simulink model "Example_Event_Separation_OB_Undirected"  (R2021b)
settings: Solver=FixedStepAuto  StartTime=0.0  StopTime=30  FixedStep=0.0001  RelTol=1e-3  EnableMultiTasking=on
values from neighbouring files (symbols this model uses):
  A = [0  1  0 ... (first row only)    [Event_Separation_OB_Undirected.m]
  ADJ = [0 1 0 0 1 0 ... (first row only)    [Event_Separation_OB_Undirected.m]
  BB = [0  0  1  0  1  0]*0    [Event_Separation_OB_Undirected.m]
  Bu = [0;0;1]    [Event_Separation_OB_Undirected.m]
  c = 1/lambda1    [Event_Separation_OB_Undirected.m]
  Cy = [1 0 0]    [Event_Separation_OB_Undirected.m]
  delta = 0.9*min(min(abs(eig(Q)))/max(abs(eig(P))),min(alpha))    [Event_Separation_OB_Undirected.m]
  F = -P*Cy'    [Event_Separation_OB_Undirected.m]
  K = -Bu'*P    [Event_Separation_OB_Undirected.m]
  LL = diag(sum(ADJ,2))-ADJ    [Event_Separation_OB_Undirected.m]
  nr = nx    [Event_Separation_OB_Undirected.m]
  nx = size(A,1)    [Event_Separation_OB_Undirected.m]
  ny = size(Cy,1)    [Event_Separation_OB_Undirected.m]
  Tc = linspace(0.11,0.16,6)    [Event_Separation_OB_Undirected.m]
  Th = 10    [Event_Separation_OB_Undirected.m]
  theta = 1    [Event_Separation_OB_Undirected.m]
  x0 = x_leader.Data    [Event_Separation_OB_Undirected.m]    (also in x0.mat = [-1.58875392951 1.07389213768 -3.08254744538 2.38426839977 -)
  x0_leader = [1 1 1]    [Event_Separation_OB_Undirected.m]
undefined symbols (not defined in the file or in its folder): Kri_m_Krj_1, Kri_m_Krj_2, Kri_m_Krj_3, Kri_m_Krj_4, Kri_m_Krj_5, Kri_m_Krj_6, ty0_1, ty0_2, ty0_3, ty0_4, ty0_5, ty0_6
settings Model: PauseTimes=0.9999  Creator=Xianwei  LastModifiedBy=kangge648
settings SolverCC: AlgebraicLoopSolver=LineSearch
settings DataIOCC: LimitDataPoints=on  ReturnWorkspaceOutputs=off
settings OptimizationCC: LifeSpan=inf
settings DebuggingCC: AllowSymbolicDim=off  SFUnexpectedBacktrackingDiag=warning  SFNoUnconditionalDefaultTransitionDiag=warning  SFExecutionAtInitializationDiag=none  SFMachineParentedDataDiag=warning  ArithmeticOperatorsInVariantConditions=warning
settings ModelReferenceCC: PropagateSignalLabelsOutOfModel=off
settings SFSimCC: SimUseLocalCustomCode=off  CustomCodeUndefinedFunction=UseInterfaceOnly
settings RTWCC: RTWUseLocalCustomCode=off
settings CodeAppCC: StateflowObjectComments=on
settings GRTTargetCC: TargetLangStandard=C89/C90 (ANSI)
settings ConfigComp: CovMetricSettings=dw  CovSaveCumulativeToWorkspaceVar=on  CovSaveSingleToWorkspaceVar=on  CovExternalEMLEnable=off

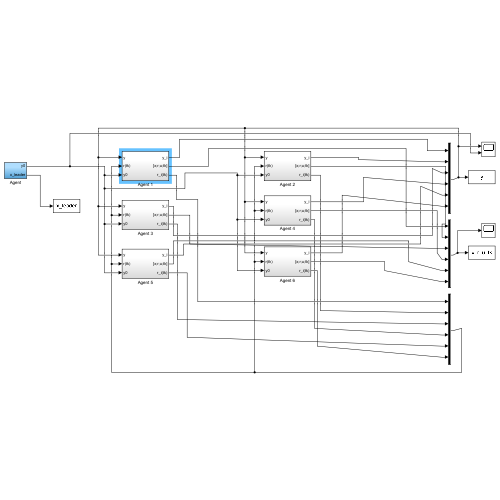
[thumbnail: Simulink's stored preview of the top-level diagram]
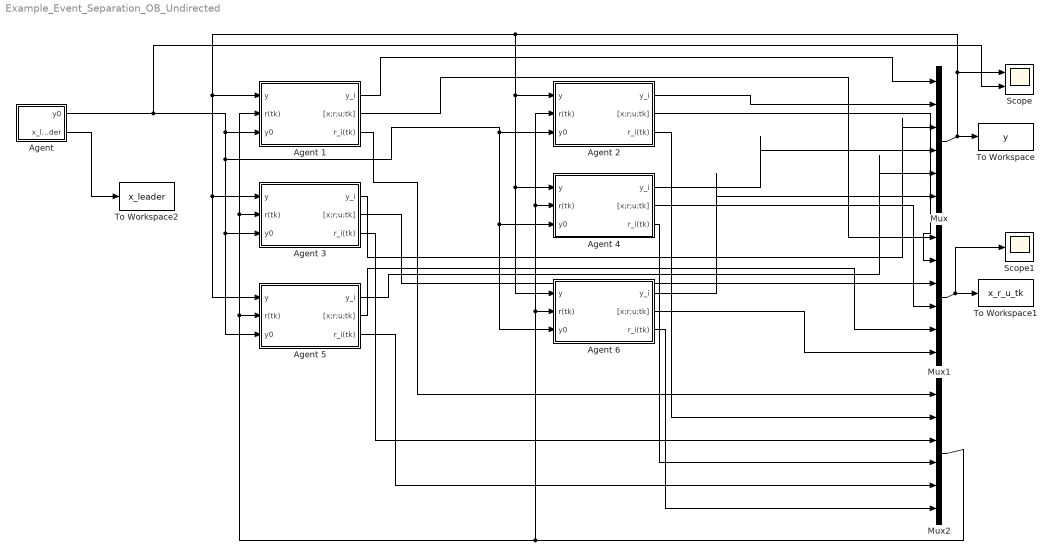
== system Example_Event_Separation_OB_Undirected ==
  Agent : Subsystem
  Agent 1 : Subsystem
  Agent 2 : Subsystem
  Agent 3 : Subsystem
  Agent 4 : Subsystem
  Agent 5 : Subsystem
  Agent 6 : Subsystem
  Mux : Mux  Inputs=6
  Mux1 : Mux  Inputs=6
  Mux2 : Mux  Inputs=6
  Scope : Scope  NumInputPorts=2
  Scope1 : Scope
  To Workspace : ToWorkspace  VariableName=y  SaveFormat=Timeseries  SampleTime=-1
  To Workspace1 : ToWorkspace  VariableName=x_r_u_tk  SaveFormat=Timeseries  SampleTime=-1
  To Workspace2 : ToWorkspace  VariableName=x_leader  SaveFormat=Timeseries  SampleTime=-1
  wires:
  Mux1/1 -> Scope1/1, To Workspace1/1
  Agent 1/1(y_i) -> Mux/1
  Agent 2/1(y_i) -> Mux/2
  Agent 3/1(y_i) -> Mux/3
  Agent 4/1(y_i) -> Mux/4
  Agent 5/1(y_i) -> Mux/5
  Agent 1/2("[x;r;u;tk]") -> Mux1/1
  Agent 2/2("[x;r;u;tk]") -> Mux1/2
  Agent 3/2("[x;r;u;tk]") -> Mux1/3
  Agent 4/2("[x;r;u;tk]") -> Mux1/4
  Agent 5/2("[x;r;u;tk]") -> Mux1/5
  Agent 1/3(r_i(tk)) -> Mux2/1
  Agent 2/3(r_i(tk)) -> Mux2/2
  Agent 3/3(r_i(tk)) -> Mux2/3
  Agent 4/3(r_i(tk)) -> Mux2/4
  Agent 5/3(r_i(tk)) -> Mux2/5
  Agent 6/3(r_i(tk)) -> Mux2/6
  Agent 6/1(y_i) -> Mux/6
  Agent 6/2("[x;r;u;tk]") -> Mux1/6
  Mux/1 -> Agent 5/1(y), Agent 3/1(y), Agent 1/1(y), Agent 6/1(y), Agent 4/1(y), Agent 2/1(y), Scope/1, To Workspace/1
  Mux2/1 -> Agent 5/2(r(tk)), Agent 3/2(r(tk)), Agent 1/2(r(tk)), Agent 6/2(r(tk)), Agent 4/2(r(tk)), Agent 2/2(r(tk))
  Agent/1(y0) -> Scope/2, Agent 6/3(y0), Agent 4/3(y0), Agent 2/3(y0), Agent 5/3(y0), Agent 3/3(y0), Agent 1/3(y0)
  Agent/2(x_leader) -> To Workspace2/1

== system Example_Event_Separation_OB_Undirected/Agent ==
  A : Gain  Gain=A  Multiplication=Matrix(K*u)
  Cy : Gain  Gain=Cy  Multiplication=Matrix(K*u)
  Integrator : Integrator  InitialCondition=x0_leader  ContinuousStateAttributes='x1'
  y0 : Outport
  x_leader : Outport  Port=2
  wires:
  Integrator/1 -> x_leader/1, A/1, Cy/1
  A/1 -> Integrator/1
  Cy/1 -> y0/1

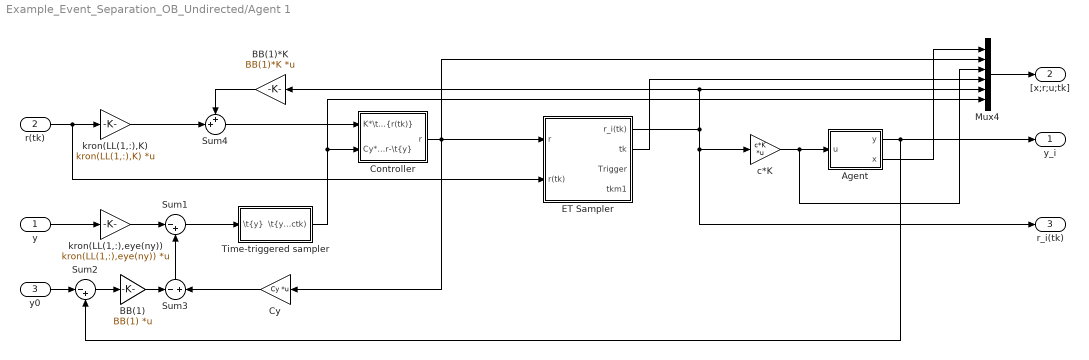
== system Example_Event_Separation_OB_Undirected/Agent 1 ==
  y : Inport
  r(tk) : Inport  Port=2
  y0 : Inport  Port=3
  Agent : Subsystem
  BB(1) : Gain  Gain=BB(1)  Multiplication=Matrix(K*u)
  BB(1)*K : Gain  Gain=BB(1)*K  Multiplication=Matrix(K*u)
  Controller : Subsystem
  Cy : Gain  Gain=Cy  Multiplication=Matrix(K*u)
  ET Sampler : Subsystem
  Mux4 : Mux  Inputs=6
  Sum1 : Sum  Inputs=|-+
  Sum2 : Sum  Inputs=|-+
  Sum3 : Sum  Inputs=-|+
  Sum4 : Sum  Inputs=++|
  Time-triggered sampler : Subsystem
  c*K : Gain  Gain=c*K  Multiplication=Matrix(K*u)
  kron(LL(1,:),K) : Gain  Gain=kron(LL(1,:),K)  Multiplication=Matrix(K*u)
  kron(LL(1,:),eye(ny)) : Gain  Gain=kron(LL(1,:),eye(ny))  Multiplication=Matrix(K*u)
  y_i : Outport
  "[x;r;u;tk]" : Outport  Port=2
  r_i(tk) : Outport  Port=3
  wires:
  Agent/2(x) -> Mux4/1
  Mux4/1 -> "[x;r;u;tk]"/1
  ET Sampler/2(tk) -> Mux4/4
  c*K/1 -> Agent/1(u), Mux4/3
  y/1 -> kron(LL(1,:),eye(ny))/1
  r(tk)/1 -> kron(LL(1,:),K)/1, ET Sampler/2(r(tk))
  kron(LL(1,:),K)/1 -> Sum4/2
  ET Sampler/1(r_i(tk)) -> BB(1)*K/1, Mux4/5, c*K/1, r_i(tk)/1
  Controller/1(r) -> Cy/1, ET Sampler/1(r), Mux4/2
  Cy/1 -> Sum3/2
  Sum1/1 -> Time-triggered sampler/1("\\t{y}")
  kron(LL(1,:),eye(ny))/1 -> Sum1/1
  Time-triggered sampler/1("\\t{y}(ctk)") -> Mux4/6, Controller/2("Cy*r-\\t{y}")
  y0/1 -> Sum2/1
  Agent/1(y) -> Sum2/2, y_i/1
  Sum2/1 -> BB(1)/1
  BB(1)/1 -> Sum3/1
  Sum3/1 -> Sum1/2
  BB(1)*K/1 -> Sum4/1
  Sum4/1 -> Controller/1("K*\\t{r(tk)}")

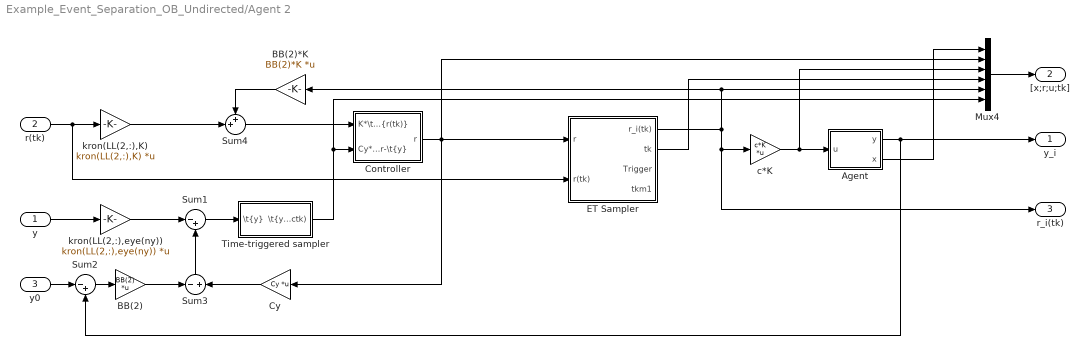
== system Example_Event_Separation_OB_Undirected/Agent 2 ==
  y : Inport
  r(tk) : Inport  Port=2
  y0 : Inport  Port=3
  Agent : Subsystem
  BB(2) : Gain  Gain=BB(2)  Multiplication=Matrix(K*u)
  BB(2)*K : Gain  Gain=BB(2)*K  Multiplication=Matrix(K*u)
  Controller : Subsystem
  Cy : Gain  Gain=Cy  Multiplication=Matrix(K*u)
  ET Sampler : Subsystem
  Mux4 : Mux  Inputs=6
  Sum1 : Sum  Inputs=|-+
  Sum2 : Sum  Inputs=|-+
  Sum3 : Sum  Inputs=-|+
  Sum4 : Sum  Inputs=++|
  Time-triggered sampler : Subsystem
  c*K : Gain  Gain=c*K  Multiplication=Matrix(K*u)
  kron(LL(2,:),K) : Gain  Gain=kron(LL(2,:),K)  Multiplication=Matrix(K*u)
  kron(LL(2,:),eye(ny)) : Gain  Gain=kron(LL(2,:),eye(ny))  Multiplication=Matrix(K*u)
  y_i : Outport
  "[x;r;u;tk]" : Outport  Port=2
  r_i(tk) : Outport  Port=3
  wires:
  c*K/1 -> Agent/1(u), Mux4/3
  r(tk)/1 -> ET Sampler/2(r(tk)), kron(LL(2,:),K)/1
  kron(LL(2,:),K)/1 -> Sum4/2
  Mux4/1 -> "[x;r;u;tk]"/1
  Controller/1(r) -> ET Sampler/1(r), Mux4/2, Cy/1
  Agent/2(x) -> Mux4/1
  kron(LL(2,:),eye(ny))/1 -> Sum1/1
  ET Sampler/2(tk) -> Mux4/4
  y/1 -> kron(LL(2,:),eye(ny))/1
  Cy/1 -> Sum3/2
  Sum1/1 -> Time-triggered sampler/1("\\t{y}")
  Time-triggered sampler/1("\\t{y}(ctk)") -> Mux4/6, Controller/2("Cy*r-\\t{y}")
  y0/1 -> Sum2/1
  Agent/1(y) -> Sum2/2, y_i/1
  BB(2)/1 -> Sum3/1
  Sum2/1 -> BB(2)/1
  Sum3/1 -> Sum1/2
  BB(2)*K/1 -> Sum4/1
  ET Sampler/1(r_i(tk)) -> BB(2)*K/1, Mux4/5, r_i(tk)/1, c*K/1
  Sum4/1 -> Controller/1("K*\\t{r(tk)}")

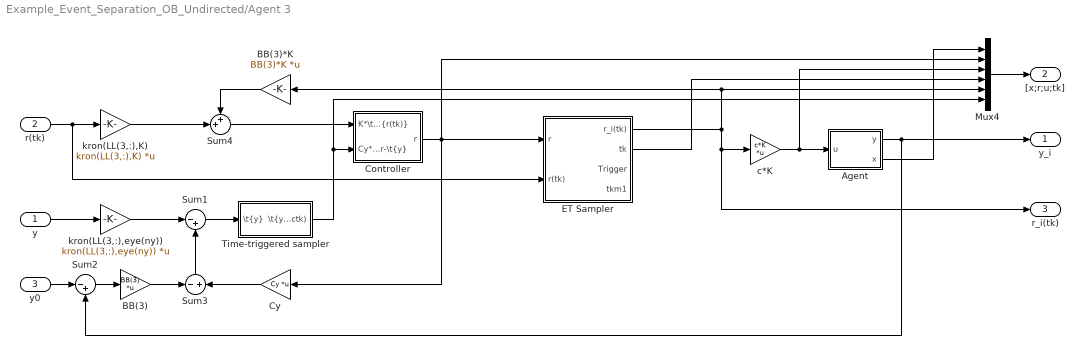
== system Example_Event_Separation_OB_Undirected/Agent 3 ==
  y : Inport
  r(tk) : Inport  Port=2
  y0 : Inport  Port=3
  Agent : Subsystem
  BB(3) : Gain  Gain=BB(3)  Multiplication=Matrix(K*u)
  BB(3)*K : Gain  Gain=BB(3)*K  Multiplication=Matrix(K*u)
  Controller : Subsystem
  Cy : Gain  Gain=Cy  Multiplication=Matrix(K*u)
  ET Sampler : Subsystem
  Mux4 : Mux  Inputs=6
  Sum1 : Sum  Inputs=|-+
  Sum2 : Sum  Inputs=|-+
  Sum3 : Sum  Inputs=-|+
  Sum4 : Sum  Inputs=++|
  Time-triggered sampler : Subsystem
  c*K : Gain  Gain=c*K  Multiplication=Matrix(K*u)
  kron(LL(3,:),K) : Gain  Gain=kron(LL(3,:),K)  Multiplication=Matrix(K*u)
  kron(LL(3,:),eye(ny)) : Gain  Gain=kron(LL(3,:),eye(ny))  Multiplication=Matrix(K*u)
  y_i : Outport
  "[x;r;u;tk]" : Outport  Port=2
  r_i(tk) : Outport  Port=3
  wires:
  c*K/1 -> Agent/1(u), Mux4/3
  r(tk)/1 -> ET Sampler/2(r(tk)), kron(LL(3,:),K)/1
  kron(LL(3,:),K)/1 -> Sum4/2
  Mux4/1 -> "[x;r;u;tk]"/1
  Controller/1(r) -> ET Sampler/1(r), Mux4/2, Cy/1
  Agent/2(x) -> Mux4/1
  kron(LL(3,:),eye(ny))/1 -> Sum1/1
  ET Sampler/2(tk) -> Mux4/4
  y/1 -> kron(LL(3,:),eye(ny))/1
  Cy/1 -> Sum3/2
  Sum1/1 -> Time-triggered sampler/1("\\t{y}")
  Time-triggered sampler/1("\\t{y}(ctk)") -> Mux4/6, Controller/2("Cy*r-\\t{y}")
  Sum2/1 -> BB(3)/1
  BB(3)/1 -> Sum3/1
  Agent/1(y) -> Sum2/2, y_i/1
  y0/1 -> Sum2/1
  Sum3/1 -> Sum1/2
  BB(3)*K/1 -> Sum4/1
  ET Sampler/1(r_i(tk)) -> BB(3)*K/1, Mux4/5, r_i(tk)/1, c*K/1
  Sum4/1 -> Controller/1("K*\\t{r(tk)}")

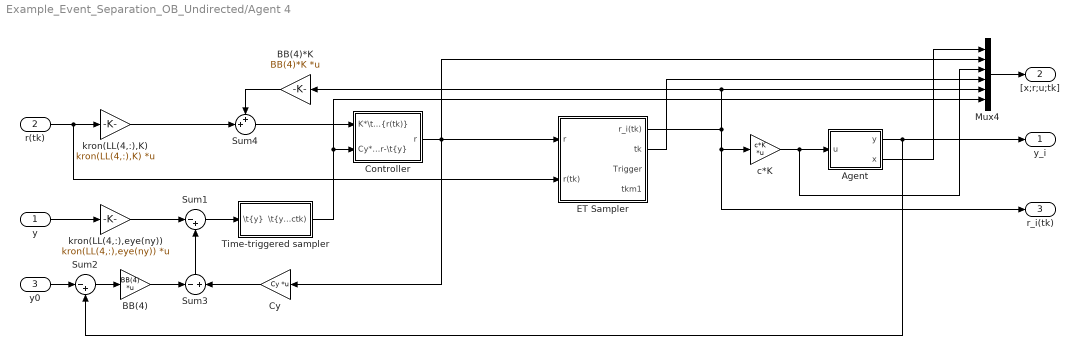
== system Example_Event_Separation_OB_Undirected/Agent 4 ==
  y : Inport
  r(tk) : Inport  Port=2
  y0 : Inport  Port=3
  Agent : Subsystem
  BB(4) : Gain  Gain=BB(4)  Multiplication=Matrix(K*u)
  BB(4)*K : Gain  Gain=BB(4)*K  Multiplication=Matrix(K*u)
  Controller : Subsystem
  Cy : Gain  Gain=Cy  Multiplication=Matrix(K*u)
  ET Sampler : Subsystem
  Mux4 : Mux  Inputs=6
  Sum1 : Sum  Inputs=|-+
  Sum2 : Sum  Inputs=|-+
  Sum3 : Sum  Inputs=-|+
  Sum4 : Sum  Inputs=++|
  Time-triggered sampler : Subsystem
  c*K : Gain  Gain=c*K  Multiplication=Matrix(K*u)
  kron(LL(4,:),K) : Gain  Gain=kron(LL(4,:),K)  Multiplication=Matrix(K*u)
  kron(LL(4,:),eye(ny)) : Gain  Gain=kron(LL(4,:),eye(ny))  Multiplication=Matrix(K*u)
  y_i : Outport
  "[x;r;u;tk]" : Outport  Port=2
  r_i(tk) : Outport  Port=3
  wires:
  y/1 -> kron(LL(4,:),eye(ny))/1
  Sum1/1 -> Time-triggered sampler/1("\\t{y}")
  Mux4/1 -> "[x;r;u;tk]"/1
  c*K/1 -> Agent/1(u), Mux4/3
  ET Sampler/2(tk) -> Mux4/4
  r(tk)/1 -> ET Sampler/2(r(tk)), kron(LL(4,:),K)/1
  Controller/1(r) -> ET Sampler/1(r), Mux4/2, Cy/1
  Agent/2(x) -> Mux4/1
  kron(LL(4,:),K)/1 -> Sum4/2
  kron(LL(4,:),eye(ny))/1 -> Sum1/1
  Time-triggered sampler/1("\\t{y}(ctk)") -> Mux4/6, Controller/2("Cy*r-\\t{y}")
  Sum2/1 -> BB(4)/1
  BB(4)/1 -> Sum3/1
  Agent/1(y) -> Sum2/2, y_i/1
  y0/1 -> Sum2/1
  Sum3/1 -> Sum1/2
  Cy/1 -> Sum3/2
  BB(4)*K/1 -> Sum4/1
  ET Sampler/1(r_i(tk)) -> BB(4)*K/1, Mux4/5, r_i(tk)/1, c*K/1
  Sum4/1 -> Controller/1("K*\\t{r(tk)}")

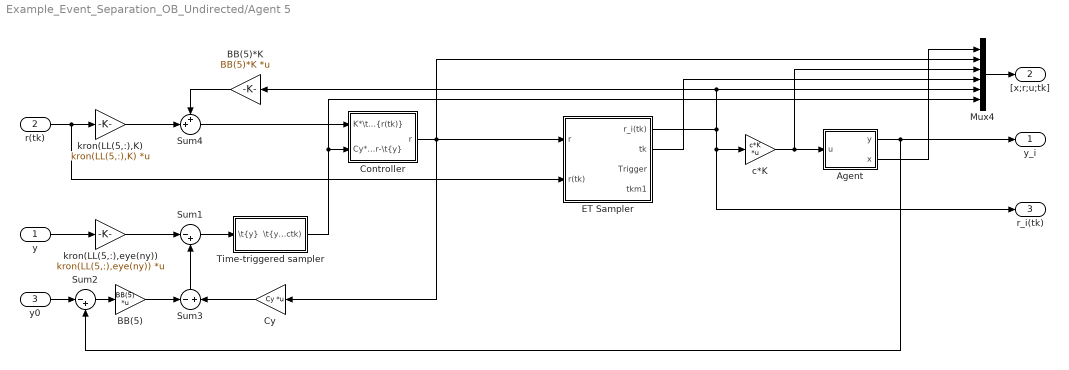
== system Example_Event_Separation_OB_Undirected/Agent 5 ==
  y : Inport
  r(tk) : Inport  Port=2
  y0 : Inport  Port=3
  Agent : Subsystem
  BB(5) : Gain  Gain=BB(5)  Multiplication=Matrix(K*u)
  BB(5)*K : Gain  Gain=BB(5)*K  Multiplication=Matrix(K*u)
  Controller : Subsystem
  Cy : Gain  Gain=Cy  Multiplication=Matrix(K*u)
  ET Sampler : Subsystem
  Mux4 : Mux  Inputs=6
  Sum1 : Sum  Inputs=|-+
  Sum2 : Sum  Inputs=|-+
  Sum3 : Sum  Inputs=-|+
  Sum4 : Sum  Inputs=++|
  Time-triggered sampler : Subsystem
  c*K : Gain  Gain=c*K  Multiplication=Matrix(K*u)
  kron(LL(5,:),K) : Gain  Gain=kron(LL(5,:),K)  Multiplication=Matrix(K*u)
  kron(LL(5,:),eye(ny)) : Gain  Gain=kron(LL(5,:),eye(ny))  Multiplication=Matrix(K*u)
  y_i : Outport
  "[x;r;u;tk]" : Outport  Port=2
  r_i(tk) : Outport  Port=3
  wires:
  kron(LL(5,:),eye(ny))/1 -> Sum1/1
  kron(LL(5,:),K)/1 -> Sum4/2
  Agent/2(x) -> Mux4/1
  Controller/1(r) -> ET Sampler/1(r), Mux4/2, Cy/1
  ET Sampler/2(tk) -> Mux4/4
  Sum1/1 -> Time-triggered sampler/1("\\t{y}")
  c*K/1 -> Agent/1(u), Mux4/3
  Mux4/1 -> "[x;r;u;tk]"/1
  r(tk)/1 -> ET Sampler/2(r(tk)), kron(LL(5,:),K)/1
  y/1 -> kron(LL(5,:),eye(ny))/1
  Time-triggered sampler/1("\\t{y}(ctk)") -> Mux4/6, Controller/2("Cy*r-\\t{y}")
  Sum2/1 -> BB(5)/1
  BB(5)/1 -> Sum3/1
  Agent/1(y) -> Sum2/2, y_i/1
  y0/1 -> Sum2/1
  Cy/1 -> Sum3/2
  Sum3/1 -> Sum1/2
  BB(5)*K/1 -> Sum4/1
  ET Sampler/1(r_i(tk)) -> Mux4/5, BB(5)*K/1, r_i(tk)/1, c*K/1
  Sum4/1 -> Controller/1("K*\\t{r(tk)}")

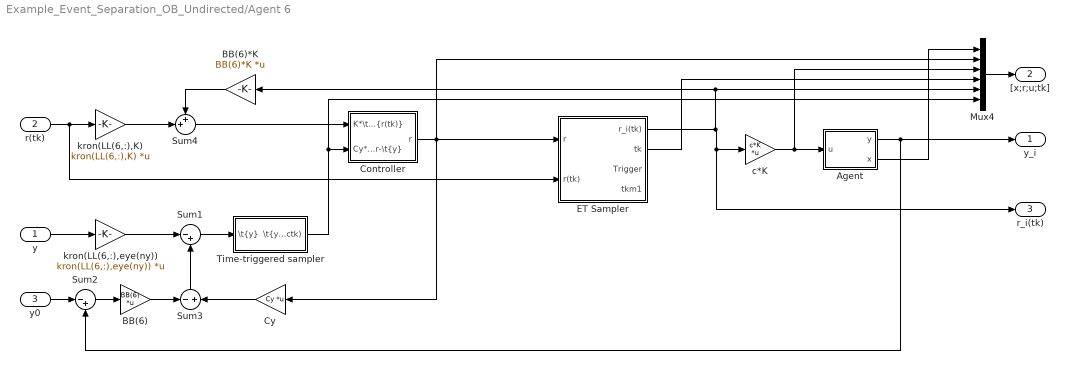
== system Example_Event_Separation_OB_Undirected/Agent 6 ==
  y : Inport
  r(tk) : Inport  Port=2
  y0 : Inport  Port=3
  Agent : Subsystem
  BB(6) : Gain  Gain=BB(6)  Multiplication=Matrix(K*u)
  BB(6)*K : Gain  Gain=BB(6)*K  Multiplication=Matrix(K*u)
  Controller : Subsystem
  Cy : Gain  Gain=Cy  Multiplication=Matrix(K*u)
  ET Sampler : Subsystem
  Mux4 : Mux  Inputs=6
  Sum1 : Sum  Inputs=|-+
  Sum2 : Sum  Inputs=|-+
  Sum3 : Sum  Inputs=-|+
  Sum4 : Sum  Inputs=++|
  Time-triggered sampler : Subsystem
  c*K : Gain  Gain=c*K  Multiplication=Matrix(K*u)
  kron(LL(6,:),K) : Gain  Gain=kron(LL(6,:),K)  Multiplication=Matrix(K*u)
  kron(LL(6,:),eye(ny)) : Gain  Gain=kron(LL(6,:),eye(ny))  Multiplication=Matrix(K*u)
  y_i : Outport
  "[x;r;u;tk]" : Outport  Port=2
  r_i(tk) : Outport  Port=3
  wires:
  r(tk)/1 -> ET Sampler/2(r(tk)), kron(LL(6,:),K)/1
  Sum1/1 -> Time-triggered sampler/1("\\t{y}")
  c*K/1 -> Agent/1(u), Mux4/3
  ET Sampler/2(tk) -> Mux4/4
  Controller/1(r) -> ET Sampler/1(r), Mux4/2, Cy/1
  Agent/2(x) -> Mux4/1
  Mux4/1 -> "[x;r;u;tk]"/1
  kron(LL(6,:),eye(ny))/1 -> Sum1/1
  y/1 -> kron(LL(6,:),eye(ny))/1
  kron(LL(6,:),K)/1 -> Sum4/2
  Time-triggered sampler/1("\\t{y}(ctk)") -> Mux4/6, Controller/2("Cy*r-\\t{y}")
  Sum2/1 -> BB(6)/1
  BB(6)/1 -> Sum3/1
  Agent/1(y) -> Sum2/2, y_i/1
  y0/1 -> Sum2/1
  Cy/1 -> Sum3/2
  Sum3/1 -> Sum1/2
  BB(6)*K/1 -> Sum4/1
  ET Sampler/1(r_i(tk)) -> Mux4/5, BB(6)*K/1, r_i(tk)/1, c*K/1
  Sum4/1 -> Controller/1("K*\\t{r(tk)}")

== system Example_Event_Separation_OB_Undirected/Agent 1/Agent ==
  u : Inport
  A : Gain  Gain=A  Multiplication=Matrix(K*u)
  Bu : Gain  Gain=Bu  Multiplication=Matrix(K*u)
  Cy : Gain  Gain=Cy  Multiplication=Matrix(K*u)
  Integrator : Integrator  InitialCondition=x0(1:nx)  ContinuousStateAttributes='x1'
  Sum5 : Sum  Inputs=|++
  y : Outport
  x : Outport  Port=2
  wires:
  Integrator/1 -> x/1, A/1, Cy/1
  A/1 -> Sum5/2
  Sum5/1 -> Integrator/1
  u/1 -> Bu/1
  Bu/1 -> Sum5/1
  Cy/1 -> y/1

== system Example_Event_Separation_OB_Undirected/Agent 1/Controller ==
  "K*\\t{r(tk)}" : Inport
  "Cy*r-\\t{y}" : Inport  Port=2
  A : Gain  Gain=A  Multiplication=Matrix(K*u)
  Bu : Gain  Gain=Bu  Multiplication=Matrix(K*u)
  F : Gain  Gain=F  Multiplication=Matrix(K*u)
  Integrator : Integrator  InitialCondition=zeros(nr,1)  ContinuousStateAttributes='r1'
  Sum5 : Sum  Inputs=+++
  c : Gain  Gain=c  Multiplication=Matrix(K*u)
  r : Outport
  wires:
  A/1 -> Sum5/3
  Sum5/1 -> Integrator/1
  Integrator/1 -> r/1, A/1
  "K*\\t{r(tk)}"/1 -> c/1
  Bu/1 -> Sum5/1
  "Cy*r-\\t{y}"/1 -> F/1
  F/1 -> Sum5/2
  c/1 -> Bu/1

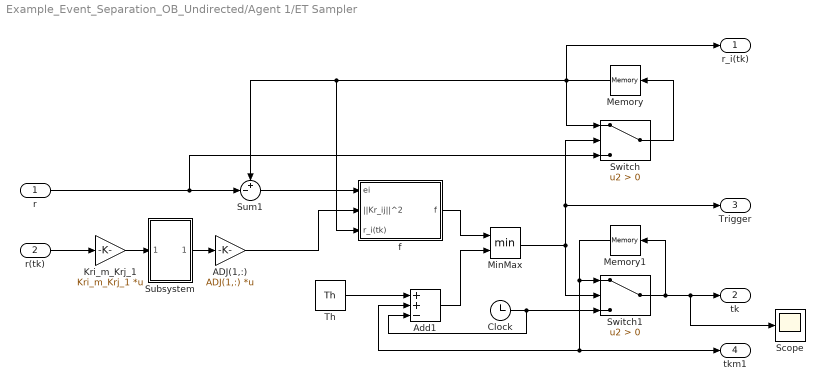
== system Example_Event_Separation_OB_Undirected/Agent 1/ET Sampler ==
  r : Inport
  r(tk) : Inport  Port=2
  ADJ(1,:) : Gain  Gain=ADJ(1,:)  Multiplication=Matrix(K*u)
  Add1 : Sum  Inputs=++-
  Clock : Clock
  Kri_m_Krj_1 : Gain  Gain=Kri_m_Krj_1  Multiplication=Matrix(K*u)
  Memory : Memory  InitialCondition=zeros(nr,1)  StateName=tilde_x
  Memory1 : Memory  StateName=tilde_x
  MinMax : MinMax  Inputs=2
  Scope : Scope
  Subsystem : Subsystem
  Sum1 : Sum  Inputs=+-|
  Switch : Switch  Criteria=u2 > Threshold
  Switch1 : Switch  Criteria=u2 > Threshold
  Th : Constant  Value=Th
  f : Subsystem
  r_i(tk) : Outport
  tk : Outport  Port=2
  Trigger : Outport  Port=3
  tkm1 : Outport  Port=4
  wires:
  Clock/1 -> Add1/3, Switch1/3
  Memory1/1 -> Switch1/1, Add1/2, tkm1/1
  Switch1/1 -> Scope/1, tk/1, Memory1/1
  Switch/1 -> Memory/1
  Sum1/1 -> f/1(ei)
  Memory/1 -> f/3(r_i(tk)), Sum1/1, r_i(tk)/1, Switch/1
  Kri_m_Krj_1/1 -> Subsystem/1(In1)
  Subsystem/1(Out1) -> ADJ(1,:)/1
  r/1 -> Sum1/2, Switch/3
  r(tk)/1 -> Kri_m_Krj_1/1
  ADJ(1,:)/1 -> f/2(||Kr_ij||^2)
  Th/1 -> Add1/1
  f/1(f) -> MinMax/1
  MinMax/1 -> Switch1/2, Trigger/1, Switch/2
  Add1/1 -> MinMax/2

== system Example_Event_Separation_OB_Undirected/Agent 1/Time-triggered sampler ==
  note: mod函数需要Tc的精度与仿真步长的精度一致，否则不能正确运算
  "\\t{y}" : Inport
  Clock : Clock
  Math Function : Math  Operator=mod  SaturateOnIntegerOverflow=on
  Memory : Memory  InitialCondition=ty0_1  StateName=tilde_x
  Scope : Scope
  Switch : Switch  Criteria=u2 > Threshold
  Tc : Constant  Value=Tc(1)
  "\\t{y}(ctk)" : Outport
  wires:
  Switch/1 -> "\\t{y}(ctk)"/1, Memory/1
  "\\t{y}"/1 -> Switch/3
  Memory/1 -> Switch/1
  Tc/1 -> Math Function/2
  Clock/1 -> Math Function/1
  Math Function/1 -> Scope/1, Switch/2

== system Example_Event_Separation_OB_Undirected/Agent 2/Agent ==
  u : Inport
  A : Gain  Gain=A  Multiplication=Matrix(K*u)
  Bu : Gain  Gain=Bu  Multiplication=Matrix(K*u)
  Cy : Gain  Gain=Cy  Multiplication=Matrix(K*u)
  Integrator : Integrator  InitialCondition=x0(nx+1:2*nx)  ContinuousStateAttributes='x1'
  Sum5 : Sum  Inputs=|++
  y : Outport
  x : Outport  Port=2
  wires:
  Integrator/1 -> x/1, A/1, Cy/1
  A/1 -> Sum5/2
  Sum5/1 -> Integrator/1
  u/1 -> Bu/1
  Bu/1 -> Sum5/1
  Cy/1 -> y/1

== system Example_Event_Separation_OB_Undirected/Agent 2/Controller ==
  "K*\\t{r(tk)}" : Inport
  "Cy*r-\\t{y}" : Inport  Port=2
  A : Gain  Gain=A  Multiplication=Matrix(K*u)
  Bu : Gain  Gain=Bu  Multiplication=Matrix(K*u)
  F : Gain  Gain=F  Multiplication=Matrix(K*u)
  Integrator : Integrator  InitialCondition=zeros(nr,1)  ContinuousStateAttributes='r1'
  Sum5 : Sum  Inputs=+++
  c : Gain  Gain=c  Multiplication=Matrix(K*u)
  r : Outport
  wires:
  A/1 -> Sum5/3
  Sum5/1 -> Integrator/1
  Integrator/1 -> r/1, A/1
  "K*\\t{r(tk)}"/1 -> c/1
  Bu/1 -> Sum5/1
  "Cy*r-\\t{y}"/1 -> F/1
  F/1 -> Sum5/2
  c/1 -> Bu/1

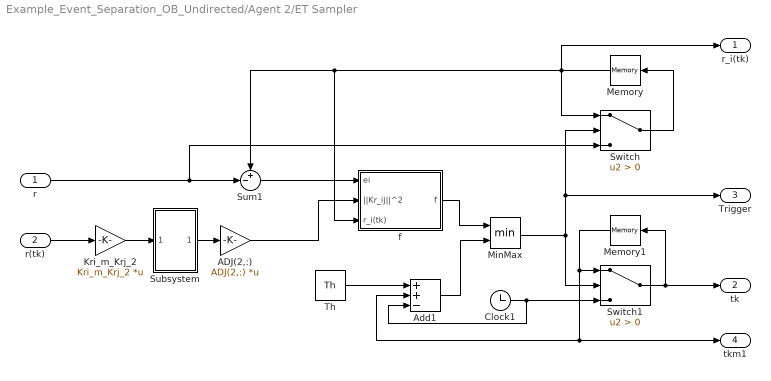
== system Example_Event_Separation_OB_Undirected/Agent 2/ET Sampler ==
  r : Inport
  r(tk) : Inport  Port=2
  ADJ(2,:) : Gain  Gain=ADJ(2,:)  Multiplication=Matrix(K*u)
  Add1 : Sum  Inputs=++-
  Clock1 : Clock
  Kri_m_Krj_2 : Gain  Gain=Kri_m_Krj_2  Multiplication=Matrix(K*u)
  Memory : Memory  InitialCondition=zeros(nr,1)  StateName=tilde_x
  Memory1 : Memory  StateName=tilde_x
  MinMax : MinMax  Inputs=2
  Subsystem : Subsystem
  Sum1 : Sum  Inputs=+-|
  Switch : Switch  Criteria=u2 > Threshold
  Switch1 : Switch  Criteria=u2 > Threshold
  Th : Constant  Value=Th
  f : Subsystem
  r_i(tk) : Outport
  tk : Outport  Port=2
  Trigger : Outport  Port=3
  tkm1 : Outport  Port=4
  wires:
  Switch/1 -> Memory/1
  Sum1/1 -> f/1(ei)
  r/1 -> Sum1/2, Switch/3
  Memory/1 -> r_i(tk)/1, Sum1/1, f/3(r_i(tk)), Switch/1
  r(tk)/1 -> Kri_m_Krj_2/1
  Kri_m_Krj_2/1 -> Subsystem/1(In1)
  Subsystem/1(Out1) -> ADJ(2,:)/1
  ADJ(2,:)/1 -> f/2(||Kr_ij||^2)
  Switch1/1 -> tk/1, Memory1/1
  MinMax/1 -> Switch1/2, Switch/2, Trigger/1
  Memory1/1 -> Switch1/1, Add1/2, tkm1/1
  Th/1 -> Add1/1
  Add1/1 -> MinMax/2
  Clock1/1 -> Switch1/3, Add1/3
  f/1(f) -> MinMax/1

== system Example_Event_Separation_OB_Undirected/Agent 2/Time-triggered sampler ==
  "\\t{y}" : Inport
  Clock : Clock
  Math Function : Math  Operator=mod  SaturateOnIntegerOverflow=on
  Memory : Memory  InitialCondition=ty0_2  StateName=tilde_x
  Switch : Switch  Criteria=u2 > Threshold
  Tc : Constant  Value=Tc(2)
  "\\t{y}(ctk)" : Outport
  wires:
  Switch/1 -> "\\t{y}(ctk)"/1, Memory/1
  "\\t{y}"/1 -> Switch/3
  Memory/1 -> Switch/1
  Tc/1 -> Math Function/2
  Clock/1 -> Math Function/1
  Math Function/1 -> Switch/2

== system Example_Event_Separation_OB_Undirected/Agent 3/Agent ==
  u : Inport
  A : Gain  Gain=A  Multiplication=Matrix(K*u)
  Bu : Gain  Gain=Bu  Multiplication=Matrix(K*u)
  Cy : Gain  Gain=Cy  Multiplication=Matrix(K*u)
  Integrator : Integrator  InitialCondition=x0(2*nx+1:3*nx)  ContinuousStateAttributes='x1'
  Sum5 : Sum  Inputs=|++
  y : Outport
  x : Outport  Port=2
  wires:
  Integrator/1 -> x/1, A/1, Cy/1
  A/1 -> Sum5/2
  Sum5/1 -> Integrator/1
  u/1 -> Bu/1
  Bu/1 -> Sum5/1
  Cy/1 -> y/1

== system Example_Event_Separation_OB_Undirected/Agent 3/Controller ==
  "K*\\t{r(tk)}" : Inport
  "Cy*r-\\t{y}" : Inport  Port=2
  A : Gain  Gain=A  Multiplication=Matrix(K*u)
  Bu : Gain  Gain=Bu  Multiplication=Matrix(K*u)
  F : Gain  Gain=F  Multiplication=Matrix(K*u)
  Integrator : Integrator  InitialCondition=zeros(nr,1)  ContinuousStateAttributes='r1'
  Sum5 : Sum  Inputs=+++
  c : Gain  Gain=c  Multiplication=Matrix(K*u)
  r : Outport
  wires:
  A/1 -> Sum5/3
  Sum5/1 -> Integrator/1
  Integrator/1 -> r/1, A/1
  "K*\\t{r(tk)}"/1 -> c/1
  Bu/1 -> Sum5/1
  "Cy*r-\\t{y}"/1 -> F/1
  F/1 -> Sum5/2
  c/1 -> Bu/1

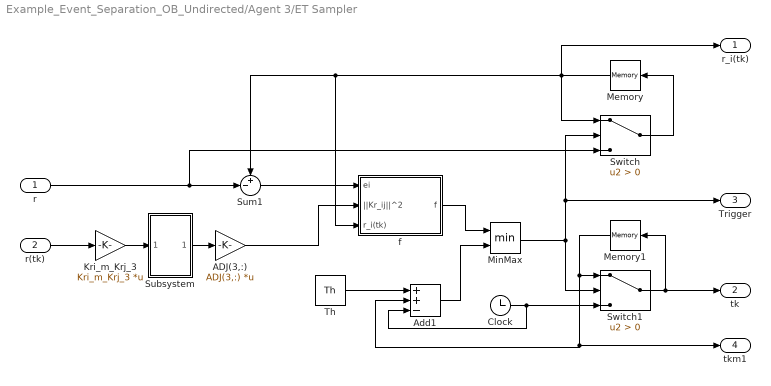
== system Example_Event_Separation_OB_Undirected/Agent 3/ET Sampler ==
  r : Inport
  r(tk) : Inport  Port=2
  ADJ(3,:) : Gain  Gain=ADJ(3,:)  Multiplication=Matrix(K*u)
  Add1 : Sum  Inputs=++-
  Clock : Clock
  Kri_m_Krj_3 : Gain  Gain=Kri_m_Krj_3  Multiplication=Matrix(K*u)
  Memory : Memory  InitialCondition=zeros(nr,1)  StateName=tilde_x
  Memory1 : Memory  StateName=tilde_x
  MinMax : MinMax  Inputs=2
  Subsystem : Subsystem
  Sum1 : Sum  Inputs=+-|
  Switch : Switch  Criteria=u2 > Threshold
  Switch1 : Switch  Criteria=u2 > Threshold
  Th : Constant  Value=Th
  f : Subsystem
  r_i(tk) : Outport
  tk : Outport  Port=2
  Trigger : Outport  Port=3
  tkm1 : Outport  Port=4
  wires:
  Switch/1 -> Memory/1
  Sum1/1 -> f/1(ei)
  r/1 -> Sum1/2, Switch/3
  Memory/1 -> Switch/1, r_i(tk)/1, f/3(r_i(tk)), Sum1/1
  r(tk)/1 -> Kri_m_Krj_3/1
  Kri_m_Krj_3/1 -> Subsystem/1(In1)
  Subsystem/1(Out1) -> ADJ(3,:)/1
  ADJ(3,:)/1 -> f/2(||Kr_ij||^2)
  Switch1/1 -> tk/1, Memory1/1
  MinMax/1 -> Switch1/2, Switch/2, Trigger/1
  Memory1/1 -> Switch1/1, Add1/2, tkm1/1
  Th/1 -> Add1/1
  Add1/1 -> MinMax/2
  Clock/1 -> Switch1/3, Add1/3
  f/1(f) -> MinMax/1

== system Example_Event_Separation_OB_Undirected/Agent 3/Time-triggered sampler ==
  "\\t{y}" : Inport
  Clock : Clock
  Math Function : Math  Operator=mod  SaturateOnIntegerOverflow=on
  Memory : Memory  InitialCondition=ty0_3  StateName=tilde_x
  Switch : Switch  Criteria=u2 > Threshold
  Tc : Constant  Value=Tc(3)
  "\\t{y}(ctk)" : Outport
  wires:
  Switch/1 -> "\\t{y}(ctk)"/1, Memory/1
  "\\t{y}"/1 -> Switch/3
  Memory/1 -> Switch/1
  Tc/1 -> Math Function/2
  Clock/1 -> Math Function/1
  Math Function/1 -> Switch/2

== system Example_Event_Separation_OB_Undirected/Agent 4/Agent ==
  u : Inport
  A : Gain  Gain=A  Multiplication=Matrix(K*u)
  Bu : Gain  Gain=Bu  Multiplication=Matrix(K*u)
  Cy : Gain  Gain=Cy  Multiplication=Matrix(K*u)
  Integrator : Integrator  InitialCondition=x0(3*nx+1:4*nx)  ContinuousStateAttributes='x1'
  Sum5 : Sum  Inputs=|++
  y : Outport
  x : Outport  Port=2
  wires:
  Integrator/1 -> x/1, A/1, Cy/1
  A/1 -> Sum5/2
  Sum5/1 -> Integrator/1
  u/1 -> Bu/1
  Bu/1 -> Sum5/1
  Cy/1 -> y/1

== system Example_Event_Separation_OB_Undirected/Agent 4/Controller ==
  "K*\\t{r(tk)}" : Inport
  "Cy*r-\\t{y}" : Inport  Port=2
  A : Gain  Gain=A  Multiplication=Matrix(K*u)
  Bu : Gain  Gain=Bu  Multiplication=Matrix(K*u)
  F : Gain  Gain=F  Multiplication=Matrix(K*u)
  Integrator : Integrator  InitialCondition=zeros(nr,1)  ContinuousStateAttributes='r1'
  Sum5 : Sum  Inputs=+++
  c : Gain  Gain=c  Multiplication=Matrix(K*u)
  r : Outport
  wires:
  A/1 -> Sum5/3
  Sum5/1 -> Integrator/1
  Integrator/1 -> r/1, A/1
  "K*\\t{r(tk)}"/1 -> c/1
  Bu/1 -> Sum5/1
  "Cy*r-\\t{y}"/1 -> F/1
  F/1 -> Sum5/2
  c/1 -> Bu/1

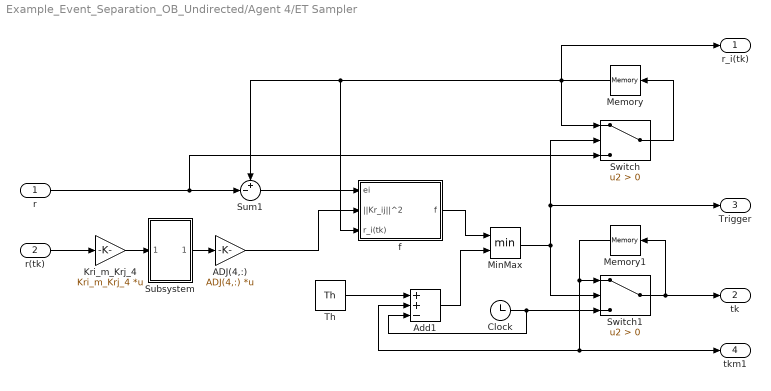
== system Example_Event_Separation_OB_Undirected/Agent 4/ET Sampler ==
  r : Inport
  r(tk) : Inport  Port=2
  ADJ(4,:) : Gain  Gain=ADJ(4,:)  Multiplication=Matrix(K*u)
  Add1 : Sum  Inputs=++-
  Clock : Clock
  Kri_m_Krj_4 : Gain  Gain=Kri_m_Krj_4  Multiplication=Matrix(K*u)
  Memory : Memory  InitialCondition=zeros(nr,1)  StateName=tilde_x
  Memory1 : Memory  StateName=tilde_x
  MinMax : MinMax  Inputs=2
  Subsystem : Subsystem
  Sum1 : Sum  Inputs=+-|
  Switch : Switch  Criteria=u2 > Threshold
  Switch1 : Switch  Criteria=u2 > Threshold
  Th : Constant  Value=Th
  f : Subsystem
  r_i(tk) : Outport
  tk : Outport  Port=2
  Trigger : Outport  Port=3
  tkm1 : Outport  Port=4
  wires:
  Switch1/1 -> tk/1, Memory1/1
  Switch/1 -> Memory/1
  Sum1/1 -> f/1(ei)
  r/1 -> Sum1/2, Switch/3
  Memory/1 -> r_i(tk)/1, f/3(r_i(tk)), Sum1/1, Switch/1
  r(tk)/1 -> Kri_m_Krj_4/1
  Kri_m_Krj_4/1 -> Subsystem/1(In1)
  Subsystem/1(Out1) -> ADJ(4,:)/1
  ADJ(4,:)/1 -> f/2(||Kr_ij||^2)
  Memory1/1 -> Switch1/1, tkm1/1, Add1/2
  Th/1 -> Add1/1
  Add1/1 -> MinMax/2
  Clock/1 -> Switch1/3, Add1/3
  f/1(f) -> MinMax/1
  MinMax/1 -> Trigger/1, Switch/2, Switch1/2

== system Example_Event_Separation_OB_Undirected/Agent 4/Time-triggered sampler ==
  "\\t{y}" : Inport
  Clock : Clock
  Math Function : Math  Operator=mod  SaturateOnIntegerOverflow=on
  Memory : Memory  InitialCondition=ty0_4  StateName=tilde_x
  Switch : Switch  Criteria=u2 > Threshold
  Tc : Constant  Value=Tc(4)
  "\\t{y}(ctk)" : Outport
  wires:
  Switch/1 -> "\\t{y}(ctk)"/1, Memory/1
  "\\t{y}"/1 -> Switch/3
  Memory/1 -> Switch/1
  Tc/1 -> Math Function/2
  Clock/1 -> Math Function/1
  Math Function/1 -> Switch/2

== system Example_Event_Separation_OB_Undirected/Agent 5/Agent ==
  u : Inport
  A : Gain  Gain=A  Multiplication=Matrix(K*u)
  Bu : Gain  Gain=Bu  Multiplication=Matrix(K*u)
  Cy : Gain  Gain=Cy  Multiplication=Matrix(K*u)
  Integrator : Integrator  InitialCondition=x0(4*nx+1:5*nx)  ContinuousStateAttributes='x1'
  Sum5 : Sum  Inputs=|++
  y : Outport
  x : Outport  Port=2
  wires:
  Integrator/1 -> x/1, A/1, Cy/1
  A/1 -> Sum5/2
  Sum5/1 -> Integrator/1
  u/1 -> Bu/1
  Bu/1 -> Sum5/1
  Cy/1 -> y/1

== system Example_Event_Separation_OB_Undirected/Agent 5/Controller ==
  "K*\\t{r(tk)}" : Inport
  "Cy*r-\\t{y}" : Inport  Port=2
  A : Gain  Gain=A  Multiplication=Matrix(K*u)
  Bu : Gain  Gain=Bu  Multiplication=Matrix(K*u)
  F : Gain  Gain=F  Multiplication=Matrix(K*u)
  Integrator : Integrator  InitialCondition=zeros(nr,1)  ContinuousStateAttributes='r1'
  Sum5 : Sum  Inputs=+++
  c : Gain  Gain=c  Multiplication=Matrix(K*u)
  r : Outport
  wires:
  A/1 -> Sum5/3
  Sum5/1 -> Integrator/1
  Integrator/1 -> r/1, A/1
  "K*\\t{r(tk)}"/1 -> c/1
  Bu/1 -> Sum5/1
  "Cy*r-\\t{y}"/1 -> F/1
  F/1 -> Sum5/2
  c/1 -> Bu/1

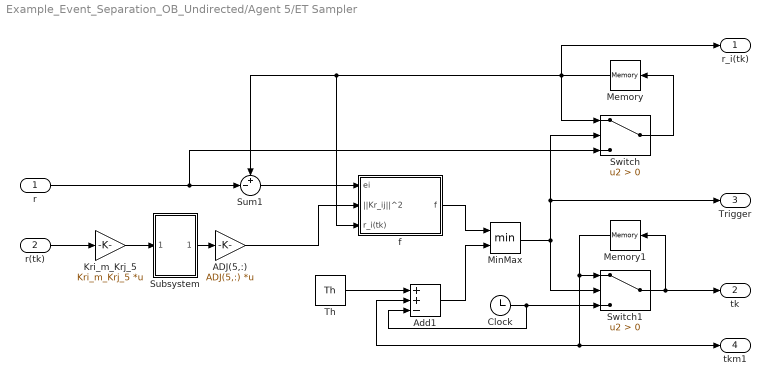
== system Example_Event_Separation_OB_Undirected/Agent 5/ET Sampler ==
  r : Inport
  r(tk) : Inport  Port=2
  ADJ(5,:) : Gain  Gain=ADJ(5,:)  Multiplication=Matrix(K*u)
  Add1 : Sum  Inputs=++-
  Clock : Clock
  Kri_m_Krj_5 : Gain  Gain=Kri_m_Krj_5  Multiplication=Matrix(K*u)
  Memory : Memory  InitialCondition=zeros(nr,1)  StateName=tilde_x
  Memory1 : Memory  StateName=tilde_x
  MinMax : MinMax  Inputs=2
  Subsystem : Subsystem
  Sum1 : Sum  Inputs=+-|
  Switch : Switch  Criteria=u2 > Threshold
  Switch1 : Switch  Criteria=u2 > Threshold
  Th : Constant  Value=Th
  f : Subsystem
  r_i(tk) : Outport
  tk : Outport  Port=2
  Trigger : Outport  Port=3
  tkm1 : Outport  Port=4
  wires:
  Switch1/1 -> tk/1, Memory1/1
  Switch/1 -> Memory/1
  Sum1/1 -> f/1(ei)
  r/1 -> Sum1/2, Switch/3
  r(tk)/1 -> Kri_m_Krj_5/1
  Kri_m_Krj_5/1 -> Subsystem/1(In1)
  Subsystem/1(Out1) -> ADJ(5,:)/1
  ADJ(5,:)/1 -> f/2(||Kr_ij||^2)
  Clock/1 -> Switch1/3, Add1/3
  Th/1 -> Add1/1
  Add1/1 -> MinMax/2
  Memory1/1 -> Switch1/1, tkm1/1, Add1/2
  MinMax/1 -> Switch1/2, Switch/2, Trigger/1
  f/1(f) -> MinMax/1
  Memory/1 -> r_i(tk)/1, f/3(r_i(tk)), Sum1/1, Switch/1

== system Example_Event_Separation_OB_Undirected/Agent 5/Time-triggered sampler ==
  "\\t{y}" : Inport
  Clock : Clock
  Math Function : Math  Operator=mod  SaturateOnIntegerOverflow=on
  Memory : Memory  InitialCondition=ty0_5  StateName=tilde_x
  Switch : Switch  Criteria=u2 > Threshold
  Tc : Constant  Value=Tc(5)
  "\\t{y}(ctk)" : Outport
  wires:
  Switch/1 -> "\\t{y}(ctk)"/1, Memory/1
  "\\t{y}"/1 -> Switch/3
  Memory/1 -> Switch/1
  Tc/1 -> Math Function/2
  Clock/1 -> Math Function/1
  Math Function/1 -> Switch/2

== system Example_Event_Separation_OB_Undirected/Agent 6/Agent ==
  u : Inport
  A : Gain  Gain=A  Multiplication=Matrix(K*u)
  Bu : Gain  Gain=Bu  Multiplication=Matrix(K*u)
  Cy : Gain  Gain=Cy  Multiplication=Matrix(K*u)
  Integrator : Integrator  InitialCondition=x0(5*nx+1:6*nx)  ContinuousStateAttributes='x1'
  Sum5 : Sum  Inputs=|++
  y : Outport
  x : Outport  Port=2
  wires:
  Integrator/1 -> x/1, A/1, Cy/1
  A/1 -> Sum5/2
  Sum5/1 -> Integrator/1
  u/1 -> Bu/1
  Bu/1 -> Sum5/1
  Cy/1 -> y/1

== system Example_Event_Separation_OB_Undirected/Agent 6/Controller ==
  "K*\\t{r(tk)}" : Inport
  "Cy*r-\\t{y}" : Inport  Port=2
  A : Gain  Gain=A  Multiplication=Matrix(K*u)
  Bu : Gain  Gain=Bu  Multiplication=Matrix(K*u)
  F : Gain  Gain=F  Multiplication=Matrix(K*u)
  Integrator : Integrator  InitialCondition=zeros(nr,1)  ContinuousStateAttributes='r1'
  Sum5 : Sum  Inputs=+++
  c : Gain  Gain=c  Multiplication=Matrix(K*u)
  r : Outport
  wires:
  A/1 -> Sum5/3
  Sum5/1 -> Integrator/1
  Integrator/1 -> r/1, A/1
  "K*\\t{r(tk)}"/1 -> c/1
  Bu/1 -> Sum5/1
  "Cy*r-\\t{y}"/1 -> F/1
  F/1 -> Sum5/2
  c/1 -> Bu/1

== system Example_Event_Separation_OB_Undirected/Agent 6/ET Sampler ==
  r : Inport
  r(tk) : Inport  Port=2
  ADJ(6,:) : Gain  Gain=ADJ(6,:)  Multiplication=Matrix(K*u)
  Add1 : Sum  Inputs=++-
  Clock : Clock
  Kri_m_Krj_6 : Gain  Gain=Kri_m_Krj_6  Multiplication=Matrix(K*u)
  Memory : Memory  InitialCondition=zeros(nr,1)  StateName=tilde_x
  Memory1 : Memory  StateName=tilde_x
  MinMax : MinMax  Inputs=2
  Subsystem : Subsystem
  Sum1 : Sum  Inputs=+-|
  Switch : Switch  Criteria=u2 > Threshold
  Switch1 : Switch  Criteria=u2 > Threshold
  Th : Constant  Value=Th
  f : Subsystem
  r_i(tk) : Outport
  tk : Outport  Port=2
  Trigger : Outport  Port=3
  tkm1 : Outport  Port=4
  wires:
  Switch1/1 -> tk/1, Memory1/1
  Switch/1 -> Memory/1
  Sum1/1 -> f/1(ei)
  r/1 -> Sum1/2, Switch/3
  Memory/1 -> r_i(tk)/1, f/3(r_i(tk)), Sum1/1, Switch/1
  r(tk)/1 -> Kri_m_Krj_6/1
  Kri_m_Krj_6/1 -> Subsystem/1(In1)
  Subsystem/1(Out1) -> ADJ(6,:)/1
  ADJ(6,:)/1 -> f/2(||Kr_ij||^2)
  Clock/1 -> Switch1/3, Add1/3
  Th/1 -> Add1/1
  Add1/1 -> MinMax/2
  Memory1/1 -> Switch1/1, Add1/2, tkm1/1
  MinMax/1 -> Switch1/2, Switch/2, Trigger/1
  f/1(f) -> MinMax/1

== system Example_Event_Separation_OB_Undirected/Agent 6/Time-triggered sampler ==
  "\\t{y}" : Inport
  Clock : Clock
  Math Function : Math  Operator=mod  SaturateOnIntegerOverflow=on
  Memory : Memory  InitialCondition=ty0_6  StateName=tilde_x
  Switch : Switch  Criteria=u2 > Threshold
  Tc : Constant  Value=Tc(6)
  "\\t{y}(ctk)" : Outport
  wires:
  Switch/1 -> "\\t{y}(ctk)"/1, Memory/1
  "\\t{y}"/1 -> Switch/3
  Memory/1 -> Switch/1
  Tc/1 -> Math Function/2
  Clock/1 -> Math Function/1
  Math Function/1 -> Switch/2

== system Example_Event_Separation_OB_Undirected/Agent 1/ET Sampler/Subsystem ==
  In1 : Inport
  Demux : Demux  Outputs=6
  Dot Product{1..6} (6 alike) : DotProduct  InputSameDT=on  OutDataTypeStr=Inherit: Inherit via internal rule
  Mux4 : Mux  Inputs=6
  Out1 : Outport
  wires:
  Demux/6 -> Dot Product5/1, Dot Product5/2
  Dot Product4/1 -> Mux4/4
  Dot Product2/1 -> Mux4/1
  Demux/1 -> Dot Product2/2, Dot Product2/1
  Demux/2 -> Dot Product3/1, Dot Product3/2
  Demux/5 -> Dot Product6/1, Dot Product6/2
  Demux/3 -> Dot Product1/1, Dot Product1/2
  Dot Product1/1 -> Mux4/3
  Demux/4 -> Dot Product4/1, Dot Product4/2
  Dot Product5/1 -> Mux4/6
  In1/1 -> Demux/1
  Dot Product6/1 -> Mux4/5
  Dot Product3/1 -> Mux4/2
  Mux4/1 -> Out1/1

== system Example_Event_Separation_OB_Undirected/Agent 1/ET Sampler/f ==
  ei : Inport
  ||Kr_ij||^2 : Inport  Port=2
  r_i(tk) : Inport  Port=3
  -delta : Gain  Gain=-delta
  2*BB(1) : Gain  Gain=2*BB(1)  Multiplication=Matrix(K*u)
  4*LL(1,1)+2*BB(1) : Gain  Gain=4*LL(1,1)+2*BB(1)  Multiplication=Matrix(K*u)
  Clock1 : Clock
  Dot Product1 : DotProduct  InputSameDT=on  OutDataTypeStr=Inherit: Inherit via internal rule
  Dot Product2 : DotProduct  InputSameDT=on  OutDataTypeStr=Inherit: Inherit via internal rule
  K : Gain  Gain=K  Multiplication=Matrix(K*u)
  K1 : Gain  Gain=K  Multiplication=Matrix(K*u)
  Math Function1 : Math  SignedPower=on  SaturateOnIntegerOverflow=on
  Sum1 : Sum  Inputs=-++
  Sum2 : Sum  Inputs=+|+
  theta : Gain  Gain=theta
  f : Outport
  wires:
  theta/1 -> Sum1/3
  Clock1/1 -> -delta/1
  ei/1 -> K/1
  K/1 -> Dot Product2/2, Dot Product2/1
  -delta/1 -> Math Function1/1
  Math Function1/1 -> theta/1
  Sum1/1 -> f/1
  Dot Product2/1 -> 4*LL(1,1)+2*BB(1)/1
  ||Kr_ij||^2/1 -> Sum2/1
  4*LL(1,1)+2*BB(1)/1 -> Sum1/1
  Dot Product1/1 -> 2*BB(1)/1
  K1/1 -> Dot Product1/2, Dot Product1/1
  r_i(tk)/1 -> K1/1
  Sum2/1 -> Sum1/2
  2*BB(1)/1 -> Sum2/2

== system Example_Event_Separation_OB_Undirected/Agent 2/ET Sampler/Subsystem ==
  In1 : Inport
  Demux : Demux  Outputs=6
  Dot Product{1..6} (6 alike) : DotProduct  InputSameDT=on  OutDataTypeStr=Inherit: Inherit via internal rule
  Mux4 : Mux  Inputs=6
  Out1 : Outport
  wires:
  Dot Product3/1 -> Mux4/2
  Demux/1 -> Dot Product2/2, Dot Product2/1
  Demux/6 -> Dot Product5/1, Dot Product5/2
  Demux/5 -> Dot Product6/1, Dot Product6/2
  Demux/4 -> Dot Product4/1, Dot Product4/2
  Demux/3 -> Dot Product1/1, Dot Product1/2
  Dot Product5/1 -> Mux4/6
  In1/1 -> Demux/1
  Dot Product6/1 -> Mux4/5
  Dot Product2/1 -> Mux4/1
  Dot Product1/1 -> Mux4/3
  Demux/2 -> Dot Product3/1, Dot Product3/2
  Dot Product4/1 -> Mux4/4
  Mux4/1 -> Out1/1

== system Example_Event_Separation_OB_Undirected/Agent 2/ET Sampler/f ==
  ei : Inport
  ||Kr_ij||^2 : Inport  Port=2
  r_i(tk) : Inport  Port=3
  -delta : Gain  Gain=-delta
  2*BB(2) : Gain  Gain=2*BB(2)  Multiplication=Matrix(K*u)
  4*LL(2,2)+2*BB(2) : Gain  Gain=4*LL(2,2)+2*BB(2)  Multiplication=Matrix(K*u)
  Clock1 : Clock
  Dot Product1 : DotProduct  InputSameDT=on  OutDataTypeStr=Inherit: Inherit via internal rule
  Dot Product2 : DotProduct  InputSameDT=on  OutDataTypeStr=Inherit: Inherit via internal rule
  K : Gain  Gain=K  Multiplication=Matrix(K*u)
  K1 : Gain  Gain=K  Multiplication=Matrix(K*u)
  Math Function1 : Math  SignedPower=on  SaturateOnIntegerOverflow=on
  Sum1 : Sum  Inputs=-++
  Sum2 : Sum  Inputs=+|+
  theta : Gain  Gain=theta
  f : Outport
  wires:
  theta/1 -> Sum1/3
  Clock1/1 -> -delta/1
  ei/1 -> K/1
  K/1 -> Dot Product2/2, Dot Product2/1
  -delta/1 -> Math Function1/1
  Math Function1/1 -> theta/1
  Sum1/1 -> f/1
  Dot Product2/1 -> 4*LL(2,2)+2*BB(2)/1
  ||Kr_ij||^2/1 -> Sum2/1
  4*LL(2,2)+2*BB(2)/1 -> Sum1/1
  K1/1 -> Dot Product1/2, Dot Product1/1
  Dot Product1/1 -> 2*BB(2)/1
  r_i(tk)/1 -> K1/1
  2*BB(2)/1 -> Sum2/2
  Sum2/1 -> Sum1/2

== system Example_Event_Separation_OB_Undirected/Agent 3/ET Sampler/Subsystem ==
  In1 : Inport
  Demux : Demux  Outputs=6
  Dot Product{1..6} (6 alike) : DotProduct  InputSameDT=on  OutDataTypeStr=Inherit: Inherit via internal rule
  Mux4 : Mux  Inputs=6
  Out1 : Outport
  wires:
  Dot Product3/1 -> Mux4/2
  Demux/1 -> Dot Product2/2, Dot Product2/1
  Demux/6 -> Dot Product5/1, Dot Product5/2
  Demux/5 -> Dot Product6/1, Dot Product6/2
  Demux/4 -> Dot Product4/1, Dot Product4/2
  Demux/3 -> Dot Product1/1, Dot Product1/2
  Dot Product5/1 -> Mux4/6
  In1/1 -> Demux/1
  Dot Product6/1 -> Mux4/5
  Dot Product2/1 -> Mux4/1
  Dot Product1/1 -> Mux4/3
  Demux/2 -> Dot Product3/1, Dot Product3/2
  Dot Product4/1 -> Mux4/4
  Mux4/1 -> Out1/1

== system Example_Event_Separation_OB_Undirected/Agent 3/ET Sampler/f ==
  ei : Inport
  ||Kr_ij||^2 : Inport  Port=2
  r_i(tk) : Inport  Port=3
  -delta : Gain  Gain=-delta
  2*BB(3) : Gain  Gain=2*BB(3)  Multiplication=Matrix(K*u)
  4*LL(3,3)+2*BB(3) : Gain  Gain=4*LL(3,3)+2*BB(3)  Multiplication=Matrix(K*u)
  Clock1 : Clock
  Dot Product1 : DotProduct  InputSameDT=on  OutDataTypeStr=Inherit: Inherit via internal rule
  Dot Product2 : DotProduct  InputSameDT=on  OutDataTypeStr=Inherit: Inherit via internal rule
  K : Gain  Gain=K  Multiplication=Matrix(K*u)
  K1 : Gain  Gain=K  Multiplication=Matrix(K*u)
  Math Function1 : Math  SignedPower=on  SaturateOnIntegerOverflow=on
  Sum1 : Sum  Inputs=-++
  Sum2 : Sum  Inputs=+|+
  theta : Gain  Gain=theta
  f : Outport
  wires:
  theta/1 -> Sum1/3
  Clock1/1 -> -delta/1
  ei/1 -> K/1
  K/1 -> Dot Product2/2, Dot Product2/1
  -delta/1 -> Math Function1/1
  Math Function1/1 -> theta/1
  Sum1/1 -> f/1
  Dot Product2/1 -> 4*LL(3,3)+2*BB(3)/1
  ||Kr_ij||^2/1 -> Sum2/1
  4*LL(3,3)+2*BB(3)/1 -> Sum1/1
  K1/1 -> Dot Product1/2, Dot Product1/1
  Dot Product1/1 -> 2*BB(3)/1
  r_i(tk)/1 -> K1/1
  2*BB(3)/1 -> Sum2/2
  Sum2/1 -> Sum1/2

== system Example_Event_Separation_OB_Undirected/Agent 4/ET Sampler/Subsystem ==
  In1 : Inport
  Demux : Demux  Outputs=6
  Dot Product{1..6} (6 alike) : DotProduct  InputSameDT=on  OutDataTypeStr=Inherit: Inherit via internal rule
  Mux4 : Mux  Inputs=6
  Out1 : Outport
  wires:
  Dot Product3/1 -> Mux4/2
  Demux/1 -> Dot Product2/2, Dot Product2/1
  Demux/6 -> Dot Product5/1, Dot Product5/2
  Demux/5 -> Dot Product6/1, Dot Product6/2
  Demux/4 -> Dot Product4/1, Dot Product4/2
  Demux/3 -> Dot Product1/1, Dot Product1/2
  Dot Product5/1 -> Mux4/6
  In1/1 -> Demux/1
  Dot Product6/1 -> Mux4/5
  Dot Product2/1 -> Mux4/1
  Dot Product1/1 -> Mux4/3
  Demux/2 -> Dot Product3/1, Dot Product3/2
  Dot Product4/1 -> Mux4/4
  Mux4/1 -> Out1/1

== system Example_Event_Separation_OB_Undirected/Agent 4/ET Sampler/f ==
  ei : Inport
  ||Kr_ij||^2 : Inport  Port=2
  r_i(tk) : Inport  Port=3
  -delta : Gain  Gain=-delta
  2*BB(4) : Gain  Gain=2*BB(4)  Multiplication=Matrix(K*u)
  4*LL(4,4)+2*BB(4) : Gain  Gain=4*LL(4,4)+2*BB(4)  Multiplication=Matrix(K*u)
  Clock1 : Clock
  Dot Product1 : DotProduct  InputSameDT=on  OutDataTypeStr=Inherit: Inherit via internal rule
  Dot Product2 : DotProduct  InputSameDT=on  OutDataTypeStr=Inherit: Inherit via internal rule
  K : Gain  Gain=K  Multiplication=Matrix(K*u)
  K1 : Gain  Gain=K  Multiplication=Matrix(K*u)
  Math Function1 : Math  SignedPower=on  SaturateOnIntegerOverflow=on
  Sum1 : Sum  Inputs=-++
  Sum2 : Sum  Inputs=+|+
  theta : Gain  Gain=theta
  f : Outport
  wires:
  theta/1 -> Sum1/3
  Clock1/1 -> -delta/1
  ei/1 -> K/1
  K/1 -> Dot Product2/2, Dot Product2/1
  -delta/1 -> Math Function1/1
  Math Function1/1 -> theta/1
  Sum1/1 -> f/1
  Dot Product2/1 -> 4*LL(4,4)+2*BB(4)/1
  ||Kr_ij||^2/1 -> Sum2/1
  4*LL(4,4)+2*BB(4)/1 -> Sum1/1
  K1/1 -> Dot Product1/2, Dot Product1/1
  Dot Product1/1 -> 2*BB(4)/1
  r_i(tk)/1 -> K1/1
  2*BB(4)/1 -> Sum2/2
  Sum2/1 -> Sum1/2

== system Example_Event_Separation_OB_Undirected/Agent 5/ET Sampler/Subsystem ==
  In1 : Inport
  Demux : Demux  Outputs=6
  Dot Product{1..6} (6 alike) : DotProduct  InputSameDT=on  OutDataTypeStr=Inherit: Inherit via internal rule
  Mux4 : Mux  Inputs=6
  Out1 : Outport
  wires:
  Dot Product3/1 -> Mux4/2
  Demux/1 -> Dot Product2/2, Dot Product2/1
  Demux/6 -> Dot Product5/1, Dot Product5/2
  Demux/5 -> Dot Product6/1, Dot Product6/2
  Demux/4 -> Dot Product4/1, Dot Product4/2
  Demux/3 -> Dot Product1/1, Dot Product1/2
  Dot Product5/1 -> Mux4/6
  In1/1 -> Demux/1
  Dot Product6/1 -> Mux4/5
  Dot Product2/1 -> Mux4/1
  Dot Product1/1 -> Mux4/3
  Demux/2 -> Dot Product3/1, Dot Product3/2
  Dot Product4/1 -> Mux4/4
  Mux4/1 -> Out1/1

== system Example_Event_Separation_OB_Undirected/Agent 5/ET Sampler/f ==
  ei : Inport
  ||Kr_ij||^2 : Inport  Port=2
  r_i(tk) : Inport  Port=3
  -delta : Gain  Gain=-delta
  2*BB(5) : Gain  Gain=2*BB(5)  Multiplication=Matrix(K*u)
  4*LL(5,5)+2*BB(5) : Gain  Gain=4*LL(5,5)+2*BB(5)  Multiplication=Matrix(K*u)
  Clock1 : Clock
  Dot Product1 : DotProduct  InputSameDT=on  OutDataTypeStr=Inherit: Inherit via internal rule
  Dot Product2 : DotProduct  InputSameDT=on  OutDataTypeStr=Inherit: Inherit via internal rule
  K : Gain  Gain=K  Multiplication=Matrix(K*u)
  K1 : Gain  Gain=K  Multiplication=Matrix(K*u)
  Math Function1 : Math  SignedPower=on  SaturateOnIntegerOverflow=on
  Sum1 : Sum  Inputs=-++
  Sum2 : Sum  Inputs=+|+
  theta : Gain  Gain=theta
  f : Outport
  wires:
  theta/1 -> Sum1/3
  Clock1/1 -> -delta/1
  ei/1 -> K/1
  K/1 -> Dot Product2/2, Dot Product2/1
  -delta/1 -> Math Function1/1
  Math Function1/1 -> theta/1
  Sum1/1 -> f/1
  Dot Product2/1 -> 4*LL(5,5)+2*BB(5)/1
  ||Kr_ij||^2/1 -> Sum2/1
  4*LL(5,5)+2*BB(5)/1 -> Sum1/1
  K1/1 -> Dot Product1/2, Dot Product1/1
  Dot Product1/1 -> 2*BB(5)/1
  r_i(tk)/1 -> K1/1
  2*BB(5)/1 -> Sum2/2
  Sum2/1 -> Sum1/2

== system Example_Event_Separation_OB_Undirected/Agent 6/ET Sampler/Subsystem ==
  In1 : Inport
  Demux : Demux  Outputs=6
  Dot Product{1..6} (6 alike) : DotProduct  InputSameDT=on  OutDataTypeStr=Inherit: Inherit via internal rule
  Mux4 : Mux  Inputs=6
  Out1 : Outport
  wires:
  Dot Product3/1 -> Mux4/2
  Demux/1 -> Dot Product2/2, Dot Product2/1
  Demux/6 -> Dot Product5/1, Dot Product5/2
  Demux/5 -> Dot Product6/1, Dot Product6/2
  Demux/4 -> Dot Product4/1, Dot Product4/2
  Demux/3 -> Dot Product1/1, Dot Product1/2
  Dot Product5/1 -> Mux4/6
  In1/1 -> Demux/1
  Dot Product6/1 -> Mux4/5
  Dot Product2/1 -> Mux4/1
  Dot Product1/1 -> Mux4/3
  Demux/2 -> Dot Product3/1, Dot Product3/2
  Dot Product4/1 -> Mux4/4
  Mux4/1 -> Out1/1

== system Example_Event_Separation_OB_Undirected/Agent 6/ET Sampler/f ==
  ei : Inport
  ||Kr_ij||^2 : Inport  Port=2
  r_i(tk) : Inport  Port=3
  -delta : Gain  Gain=-delta
  2*BB(6) : Gain  Gain=2*BB(6)  Multiplication=Matrix(K*u)
  4*LL(6,6)+2*BB(6) : Gain  Gain=4*LL(6,6)+2*BB(6)  Multiplication=Matrix(K*u)
  Clock1 : Clock
  Dot Product1 : DotProduct  InputSameDT=on  OutDataTypeStr=Inherit: Inherit via internal rule
  Dot Product2 : DotProduct  InputSameDT=on  OutDataTypeStr=Inherit: Inherit via internal rule
  K : Gain  Gain=K  Multiplication=Matrix(K*u)
  K1 : Gain  Gain=K  Multiplication=Matrix(K*u)
  Math Function1 : Math  SignedPower=on  SaturateOnIntegerOverflow=on
  Sum1 : Sum  Inputs=-++
  Sum2 : Sum  Inputs=+|+
  theta : Gain  Gain=theta
  f : Outport
  wires:
  theta/1 -> Sum1/3
  Clock1/1 -> -delta/1
  ei/1 -> K/1
  K/1 -> Dot Product2/2, Dot Product2/1
  -delta/1 -> Math Function1/1
  Math Function1/1 -> theta/1
  Sum1/1 -> f/1
  Dot Product2/1 -> 4*LL(6,6)+2*BB(6)/1
  ||Kr_ij||^2/1 -> Sum2/1
  4*LL(6,6)+2*BB(6)/1 -> Sum1/1
  K1/1 -> Dot Product1/2, Dot Product1/1
  Dot Product1/1 -> 2*BB(6)/1
  r_i(tk)/1 -> K1/1
  2*BB(6)/1 -> Sum2/2
  Sum2/1 -> Sum1/2
